simulink model "kinematics20221024"  (R2020a)
settings: Solver=VariableStepAuto  StartTime=0.0  StopTime=12  FixedStep=0.01  RelTol=1e-3
undefined symbols (not defined in the file or in its folder): X, Y, Z
libraries: sm_lib x198, nesl_utility x61, sm_cable_robot_lib x44, simulink x1
(part 8 of 8)

== system kinematics20221024/Frame2/Column 1/Lower Motor Assembly/Motor/Double Bracket ==
  Base Center Frame : sm_lib/Frames and Transforms/Reference Frame
  Left Bracket : sm_cable_robot_lib/Bracket  height=height  width=width  thickness=thickness  holeOffset=holeOffset  holeRadius=holeRadius  rho=rho  color=color
      settings: SourceProductBaseCode=MS
  Left Bracket xForm : sm_lib/Frames and Transforms/Rigid Transform  TranslationMethod=StandardAxis  TranslationStandardOffset=0.5*offset  TranslationLengthUnit=m  TranslationStandardAxis=-Y  TranslationCartesianOffset=[0 0 0]  TranslationROffset=0  TranslationROffsetUnits=m  TranslationZOffset=0  TranslationZOffsetUnits=m  TranslationThetaOffset=0  TranslationThetaOffsetUnits=deg  RotationMethod=AlignedAxes  RotationAngleUnits=deg  RotationStandardAxis=+X  RotationAngle=90  RotationArbitraryAxis=[0 0 1]  FollAlignAxisA=+X  BaseAlignAxisA=+X  FollAlignAxisB=+Y  BaseAlignAxisB=+Z  RotationSequenceAxes=FollowerAxes  RotationSequence=XYX  RotationSequenceAngles=[0 0 0]  RotationSequenceAnglesUnits=deg  RotationMatrix=[1 0 0; 0 1 0; 0 0 1]
  Right Bracket : sm_cable_robot_lib/Bracket  height=height  width=width  thickness=thickness  holeOffset=holeOffset  holeRadius=holeRadius  rho=rho  color=color
      settings: SourceProductBaseCode=MS
  Right Bracket xForm : sm_lib/Frames and Transforms/Rigid Transform  TranslationMethod=StandardAxis  TranslationStandardOffset=0.5*offset  TranslationLengthUnit=m  TranslationStandardAxis=+Y  TranslationCartesianOffset=[0 0 0]  TranslationROffset=0  TranslationROffsetUnits=m  TranslationZOffset=0  TranslationZOffsetUnits=m  TranslationThetaOffset=0  TranslationThetaOffsetUnits=deg  RotationMethod=AlignedAxes  RotationAngleUnits=deg  RotationStandardAxis=+X  RotationAngle=90  RotationArbitraryAxis=[0 0 1]  FollAlignAxisA=+X  BaseAlignAxisA=+X  FollAlignAxisB=+Y  BaseAlignAxisB=+Z  RotationSequenceAxes=FollowerAxes  RotationSequence=XYX  RotationSequenceAngles=[0 0 0]  RotationSequenceAnglesUnits=deg  RotationMatrix=[1 0 0; 0 1 0; 0 0 1]
  B : PMIOPort  Side=Left
  connections:
  B/RConn1 -- Base Center Frame/RConn1 -- Right Bracket xForm/LConn1 -- Left Bracket xForm/LConn1
  Right Bracket/LConn1 -- Right Bracket xForm/RConn1
  Left Bracket/LConn1 -- Left Bracket xForm/RConn1

== system kinematics20221024/Frame2/Column 2/Lower Motor Assembly1/Motor/Double Bracket ==
  Base Center Frame : sm_lib/Frames and Transforms/Reference Frame
  Left Bracket : sm_cable_robot_lib/Bracket  height=height  width=width  thickness=thickness  holeOffset=holeOffset  holeRadius=holeRadius  rho=rho  color=color
      settings: SourceProductBaseCode=MS
  Left Bracket xForm : sm_lib/Frames and Transforms/Rigid Transform  TranslationMethod=StandardAxis  TranslationStandardOffset=0.5*offset  TranslationLengthUnit=m  TranslationStandardAxis=-Y  TranslationCartesianOffset=[0 0 0]  TranslationROffset=0  TranslationROffsetUnits=m  TranslationZOffset=0  TranslationZOffsetUnits=m  TranslationThetaOffset=0  TranslationThetaOffsetUnits=deg  RotationMethod=AlignedAxes  RotationAngleUnits=deg  RotationStandardAxis=+X  RotationAngle=90  RotationArbitraryAxis=[0 0 1]  FollAlignAxisA=+X  BaseAlignAxisA=+X  FollAlignAxisB=+Y  BaseAlignAxisB=+Z  RotationSequenceAxes=FollowerAxes  RotationSequence=XYX  RotationSequenceAngles=[0 0 0]  RotationSequenceAnglesUnits=deg  RotationMatrix=[1 0 0; 0 1 0; 0 0 1]
  Right Bracket : sm_cable_robot_lib/Bracket  height=height  width=width  thickness=thickness  holeOffset=holeOffset  holeRadius=holeRadius  rho=rho  color=color
      settings: SourceProductBaseCode=MS
  Right Bracket xForm : sm_lib/Frames and Transforms/Rigid Transform  TranslationMethod=StandardAxis  TranslationStandardOffset=0.5*offset  TranslationLengthUnit=m  TranslationStandardAxis=+Y  TranslationCartesianOffset=[0 0 0]  TranslationROffset=0  TranslationROffsetUnits=m  TranslationZOffset=0  TranslationZOffsetUnits=m  TranslationThetaOffset=0  TranslationThetaOffsetUnits=deg  RotationMethod=AlignedAxes  RotationAngleUnits=deg  RotationStandardAxis=+X  RotationAngle=90  RotationArbitraryAxis=[0 0 1]  FollAlignAxisA=+X  BaseAlignAxisA=+X  FollAlignAxisB=+Y  BaseAlignAxisB=+Z  RotationSequenceAxes=FollowerAxes  RotationSequence=XYX  RotationSequenceAngles=[0 0 0]  RotationSequenceAnglesUnits=deg  RotationMatrix=[1 0 0; 0 1 0; 0 0 1]
  B : PMIOPort  Side=Left
  connections:
  B/RConn1 -- Base Center Frame/RConn1 -- Right Bracket xForm/LConn1 -- Left Bracket xForm/LConn1
  Right Bracket/LConn1 -- Right Bracket xForm/RConn1
  Left Bracket/LConn1 -- Left Bracket xForm/RConn1

== system kinematics20221024/Frame2/Column 3/Lower Motor Assembly/Motor/Double Bracket ==
  Base Center Frame : sm_lib/Frames and Transforms/Reference Frame
  Left Bracket : sm_cable_robot_lib/Bracket  height=height  width=width  thickness=thickness  holeOffset=holeOffset  holeRadius=holeRadius  rho=rho  color=color
      settings: SourceProductBaseCode=MS
  Left Bracket xForm : sm_lib/Frames and Transforms/Rigid Transform  TranslationMethod=StandardAxis  TranslationStandardOffset=0.5*offset  TranslationLengthUnit=m  TranslationStandardAxis=-Y  TranslationCartesianOffset=[0 0 0]  TranslationROffset=0  TranslationROffsetUnits=m  TranslationZOffset=0  TranslationZOffsetUnits=m  TranslationThetaOffset=0  TranslationThetaOffsetUnits=deg  RotationMethod=AlignedAxes  RotationAngleUnits=deg  RotationStandardAxis=+X  RotationAngle=90  RotationArbitraryAxis=[0 0 1]  FollAlignAxisA=+X  BaseAlignAxisA=+X  FollAlignAxisB=+Y  BaseAlignAxisB=+Z  RotationSequenceAxes=FollowerAxes  RotationSequence=XYX  RotationSequenceAngles=[0 0 0]  RotationSequenceAnglesUnits=deg  RotationMatrix=[1 0 0; 0 1 0; 0 0 1]
  Right Bracket : sm_cable_robot_lib/Bracket  height=height  width=width  thickness=thickness  holeOffset=holeOffset  holeRadius=holeRadius  rho=rho  color=color
      settings: SourceProductBaseCode=MS
  Right Bracket xForm : sm_lib/Frames and Transforms/Rigid Transform  TranslationMethod=StandardAxis  TranslationStandardOffset=0.5*offset  TranslationLengthUnit=m  TranslationStandardAxis=+Y  TranslationCartesianOffset=[0 0 0]  TranslationROffset=0  TranslationROffsetUnits=m  TranslationZOffset=0  TranslationZOffsetUnits=m  TranslationThetaOffset=0  TranslationThetaOffsetUnits=deg  RotationMethod=AlignedAxes  RotationAngleUnits=deg  RotationStandardAxis=+X  RotationAngle=90  RotationArbitraryAxis=[0 0 1]  FollAlignAxisA=+X  BaseAlignAxisA=+X  FollAlignAxisB=+Y  BaseAlignAxisB=+Z  RotationSequenceAxes=FollowerAxes  RotationSequence=XYX  RotationSequenceAngles=[0 0 0]  RotationSequenceAnglesUnits=deg  RotationMatrix=[1 0 0; 0 1 0; 0 0 1]
  B : PMIOPort  Side=Left
  connections:
  B/RConn1 -- Base Center Frame/RConn1 -- Right Bracket xForm/LConn1 -- Left Bracket xForm/LConn1
  Right Bracket/LConn1 -- Right Bracket xForm/RConn1
  Left Bracket/LConn1 -- Left Bracket xForm/RConn1

== system kinematics20221024/Frame2/Column 4/Lower Motor Assembly/Motor/Double Bracket ==
  Base Center Frame : sm_lib/Frames and Transforms/Reference Frame
  Left Bracket : sm_cable_robot_lib/Bracket  height=height  width=width  thickness=thickness  holeOffset=holeOffset  holeRadius=holeRadius  rho=rho  color=color
      settings: SourceProductBaseCode=MS
  Left Bracket xForm : sm_lib/Frames and Transforms/Rigid Transform  TranslationMethod=StandardAxis  TranslationStandardOffset=0.5*offset  TranslationLengthUnit=m  TranslationStandardAxis=-Y  TranslationCartesianOffset=[0 0 0]  TranslationROffset=0  TranslationROffsetUnits=m  TranslationZOffset=0  TranslationZOffsetUnits=m  TranslationThetaOffset=0  TranslationThetaOffsetUnits=deg  RotationMethod=AlignedAxes  RotationAngleUnits=deg  RotationStandardAxis=+X  RotationAngle=90  RotationArbitraryAxis=[0 0 1]  FollAlignAxisA=+X  BaseAlignAxisA=+X  FollAlignAxisB=+Y  BaseAlignAxisB=+Z  RotationSequenceAxes=FollowerAxes  RotationSequence=XYX  RotationSequenceAngles=[0 0 0]  RotationSequenceAnglesUnits=deg  RotationMatrix=[1 0 0; 0 1 0; 0 0 1]
  Right Bracket : sm_cable_robot_lib/Bracket  height=height  width=width  thickness=thickness  holeOffset=holeOffset  holeRadius=holeRadius  rho=rho  color=color
      settings: SourceProductBaseCode=MS
  Right Bracket xForm : sm_lib/Frames and Transforms/Rigid Transform  TranslationMethod=StandardAxis  TranslationStandardOffset=0.5*offset  TranslationLengthUnit=m  TranslationStandardAxis=+Y  TranslationCartesianOffset=[0 0 0]  TranslationROffset=0  TranslationROffsetUnits=m  TranslationZOffset=0  TranslationZOffsetUnits=m  TranslationThetaOffset=0  TranslationThetaOffsetUnits=deg  RotationMethod=AlignedAxes  RotationAngleUnits=deg  RotationStandardAxis=+X  RotationAngle=90  RotationArbitraryAxis=[0 0 1]  FollAlignAxisA=+X  BaseAlignAxisA=+X  FollAlignAxisB=+Y  BaseAlignAxisB=+Z  RotationSequenceAxes=FollowerAxes  RotationSequence=XYX  RotationSequenceAngles=[0 0 0]  RotationSequenceAnglesUnits=deg  RotationMatrix=[1 0 0; 0 1 0; 0 0 1]
  B : PMIOPort  Side=Left
  connections:
  B/RConn1 -- Base Center Frame/RConn1 -- Right Bracket xForm/LConn1 -- Left Bracket xForm/LConn1
  Right Bracket/LConn1 -- Right Bracket xForm/RConn1
  Left Bracket/LConn1 -- Left Bracket xForm/RConn1
